simulink model "Demo"  (R2019a)
settings: Solver=VariableStepAuto  StartTime=0.0  StopTime=10.0  FixedStep=10e-6  RelTol=1e-3
StopFcn:
  | run PlotResults.m
settings Model: Creator=visha  LastModifiedBy=visha
settings SolverCC: AlgebraicLoopSolver=LineSearch

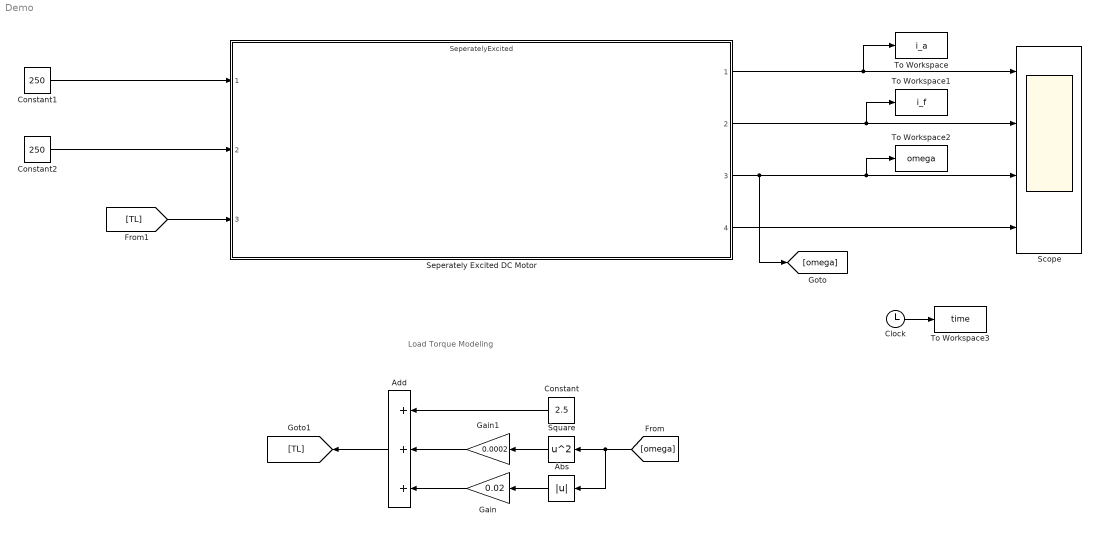
== system Demo ==
  note: Load Torque Modeling
  Abs : Abs
  Add : Sum  Inputs=+++
  Clock : Clock
  Constant : Constant  Value=2.5
  Constant1 : Constant  Value=250
  Constant2 : Constant  Value=250
  Gain : Gain  Gain=0.02
  Gain1 : Gain  Gain=0.0002
  Scope : Scope  NumInputPorts=4
  "Seperately Excited DC Motor " : ModelReference  ModelNameDialog=SeperatelyExcited.slx  SimulationMode=Normal  ModelReferenceVersion=1.15
  Square : Math  Operator=square  SaturateOnIntegerOverflow=on
  To Workspace : ToWorkspace  VariableName=i_a  SaveFormat=Timeseries  SampleTime=-1
  To Workspace1 : ToWorkspace  VariableName=i_f  SaveFormat=Timeseries  SampleTime=-1
  To Workspace2 : ToWorkspace  VariableName=omega  SaveFormat=Timeseries  SampleTime=-1
  To Workspace3 : ToWorkspace  VariableName=time  SaveFormat=Timeseries  SampleTime=-1
  wires:
  Square/1 -> Gain1/1
  Abs/1 -> Gain/1
  Gain/1 -> Add/3
  Gain1/1 -> Add/2
  Constant/1 -> Add/1
  [omega] -> Abs/1, Square/1
  "Seperately Excited DC Motor "/3 -> To Workspace2/1, Scope/3, [omega]
  Add/1 -> [TL]
  [TL] -> "Seperately Excited DC Motor "/3
  Constant2/1 -> "Seperately Excited DC Motor "/2
  Constant1/1 -> "Seperately Excited DC Motor "/1
  "Seperately Excited DC Motor "/1 -> To Workspace/1, Scope/1
  "Seperately Excited DC Motor "/2 -> To Workspace1/1, Scope/2
  "Seperately Excited DC Motor "/4 -> Scope/4
  Clock/1 -> To Workspace3/1
